simulink model "vd_controller"  (R2019b)
settings: configuration reference "E9_ECU_Configuration" (kept outside this file)
undefined symbols (not defined in the file or in its folder): BrakeMap_default_breakpoints, BrakeMap_default_data, disable_9D_front, disable_slipanglesensor, mask_select_input_pGL, Sq_PosBadGradient, Sq_PosIsFrozen, Sq_PosOutOfBounds
libraries: SignalProcessingSensorFusionLib x38, simulink x30, hdlsllib x3
(part 2 of 2)

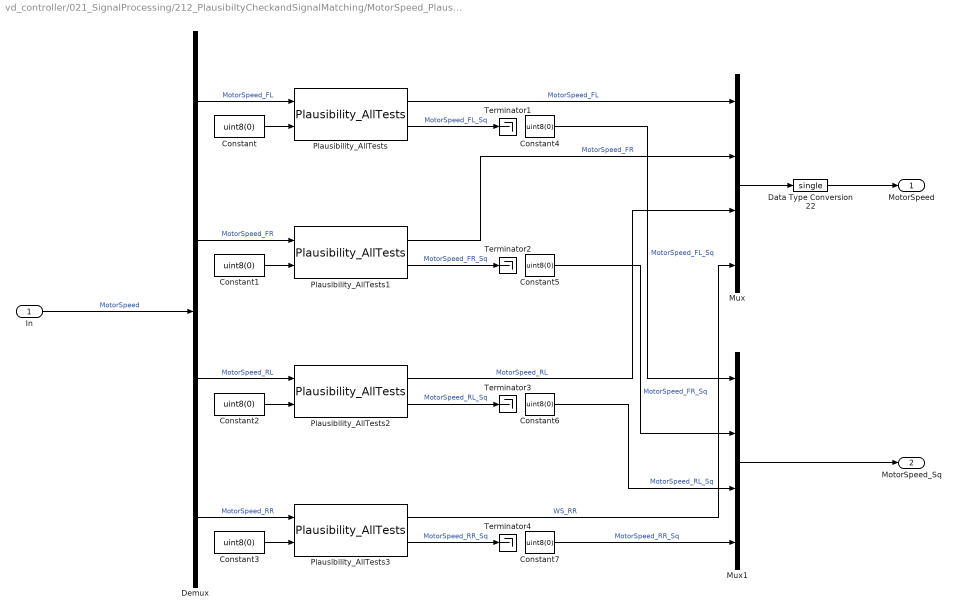
== system vd_controller/021_SignalProcessing/212_PlausibiltyCheckandSignalMatching/MotorSpeed_Plausibility ==
  In : Inport
  Constant{,1..7} (8 alike) : Constant  Value=uint8(0)
  Data Type Conversion22 : DataTypeConversion  OutDataTypeStr=single
  Demux : Demux
  Mux : Mux
  Mux1 : Mux
  Plausibility_AllTests : SignalProcessingSensorFusionLib/Plausibility_AllTests  alpha=0.4  checkGradient=off  deviation=0  threshold=0  alpha2=0  increasingPercentage=0  signalBounds=1e-10  stepDelay=40  upperBound=20000  lowerBound=-10000  useAlternativeValue=off  useManualAlternativeValue=off  manualAlternativeValue=0
  Plausibility_AllTests1 : SignalProcessingSensorFusionLib/Plausibility_AllTests  alpha=0.4  checkGradient=off  deviation=0  threshold=0  alpha2=0  increasingPercentage=0  signalBounds=1e-10  stepDelay=40  upperBound=20000  lowerBound=-10000  useAlternativeValue=off  useManualAlternativeValue=off  manualAlternativeValue=0
  Plausibility_AllTests2 : SignalProcessingSensorFusionLib/Plausibility_AllTests  alpha=0.4  checkGradient=off  deviation=0  threshold=0  alpha2=0  increasingPercentage=0  signalBounds=1e-10  stepDelay=40  upperBound=20000  lowerBound=-10000  useAlternativeValue=off  useManualAlternativeValue=off  manualAlternativeValue=0
  Plausibility_AllTests3 : SignalProcessingSensorFusionLib/Plausibility_AllTests  alpha=0  checkGradient=off  deviation=0  threshold=0  alpha2=0  increasingPercentage=0  signalBounds=1e-10  stepDelay=40  upperBound=20000  lowerBound=-10000  useAlternativeValue=off  useManualAlternativeValue=off  manualAlternativeValue=0
  Terminator{1..4} (4 alike) : Terminator
  MotorSpeed : Outport  VectorParamsAs1DForOutWhenUnconnected=off
  MotorSpeed_Sq : Outport  Port=2  VectorParamsAs1DForOutWhenUnconnected=off
  wires:
  Constant4/1 -> Mux1/1  "MotorSpeed_FL_Sq"
  Constant7/1 -> Mux1/4  "MotorSpeed_RR_Sq"
  Mux1/1 -> MotorSpeed_Sq/1
  Mux/1 -> Data Type Conversion22/1
  Plausibility_AllTests3/1 -> Mux/4  "WS_RR"
  Constant3/1 -> Plausibility_AllTests3/2
  Constant2/1 -> Plausibility_AllTests2/2
  Constant1/1 -> Plausibility_AllTests1/2
  Constant/1 -> Plausibility_AllTests/2
  Demux/4 -> Plausibility_AllTests3/1  "MotorSpeed_RR"
  Constant5/1 -> Mux1/2  "MotorSpeed_FR_Sq"
  Constant6/1 -> Mux1/3  "MotorSpeed_RL_Sq"
  Demux/3 -> Plausibility_AllTests2/1  "MotorSpeed_RL"
  Demux/2 -> Plausibility_AllTests1/1  "MotorSpeed_FR"
  Demux/1 -> Plausibility_AllTests/1  "MotorSpeed_FL"
  Plausibility_AllTests2/1 -> Mux/3  "MotorSpeed_RL"
  Plausibility_AllTests/1 -> Mux/1  "MotorSpeed_FL"
  In/1 -> Demux/1  "MotorSpeed"
  Plausibility_AllTests1/1 -> Mux/2  "MotorSpeed_FR"
  Data Type Conversion22/1 -> MotorSpeed/1
  Plausibility_AllTests/2 -> Terminator1/1  "MotorSpeed_FL_Sq"
  Plausibility_AllTests1/2 -> Terminator2/1  "MotorSpeed_FR_Sq"
  Plausibility_AllTests2/2 -> Terminator3/1  "MotorSpeed_RL_Sq"
  Plausibility_AllTests3/2 -> Terminator4/1  "MotorSpeed_RR_Sq"

== system vd_controller/021_SignalProcessing/212_PlausibiltyCheckandSignalMatching/MotorTemp_Plausibility ==
  In : Inport
  Constant{,1..3} (4 alike) : Constant  Value=uint8(0)
  Data Type Conversion{1..3,22} (4 alike) : DataTypeConversion  OutDataTypeStr=single
  Demux : Demux
  Mux : Mux
  Mux1 : Mux
  Plausibility_AllTests{,1..3} (4 alike) : SignalProcessingSensorFusionLib/Plausibility_AllTests  alpha=0.5  checkGradient=off  deviation=0  threshold=0  alpha2=0  increasingPercentage=0  signalBounds=1e-12  stepDelay=40  upperBound=250  lowerBound=-10  useAlternativeValue=off  useManualAlternativeValue=off  manualAlternativeValue=0
  MotorTempPlausible : Outport  VectorParamsAs1DForOutWhenUnconnected=off
  MotorTemp_Sq : Outport  Port=2  VectorParamsAs1DForOutWhenUnconnected=off
  wires:
  Plausibility_AllTests1/1 -> Data Type Conversion1/1  "MotorTemp_FR"
  In/1 -> Demux/1  "motorTemp"
  Plausibility_AllTests/1 -> Data Type Conversion22/1  "MotorTemp_FL"
  Plausibility_AllTests2/1 -> Data Type Conversion2/1  "MotorTemp_RL"
  Demux/1 -> Plausibility_AllTests/1
  Demux/2 -> Plausibility_AllTests1/1
  Demux/3 -> Plausibility_AllTests2/1
  Plausibility_AllTests2/2 -> Mux1/3  "MotorTemp_RL_Sq"
  Plausibility_AllTests1/2 -> Mux1/2  "MotorTemp_FR_Sq"
  Demux/4 -> Plausibility_AllTests3/1
  Constant/1 -> Plausibility_AllTests/2
  Constant1/1 -> Plausibility_AllTests1/2
  Constant2/1 -> Plausibility_AllTests2/2
  Constant3/1 -> Plausibility_AllTests3/2
  Plausibility_AllTests3/1 -> Data Type Conversion3/1  "MotorTemp_RR"
  Mux/1 -> MotorTempPlausible/1
  Mux1/1 -> MotorTemp_Sq/1
  Plausibility_AllTests3/2 -> Mux1/4  "MotorTemp_RR_Sq"
  Plausibility_AllTests/2 -> Mux1/1  "MotorTemp_Sq"
  Data Type Conversion22/1 -> Mux/1
  Data Type Conversion1/1 -> Mux/2
  Data Type Conversion2/1 -> Mux/3
  Data Type Conversion3/1 -> Mux/4

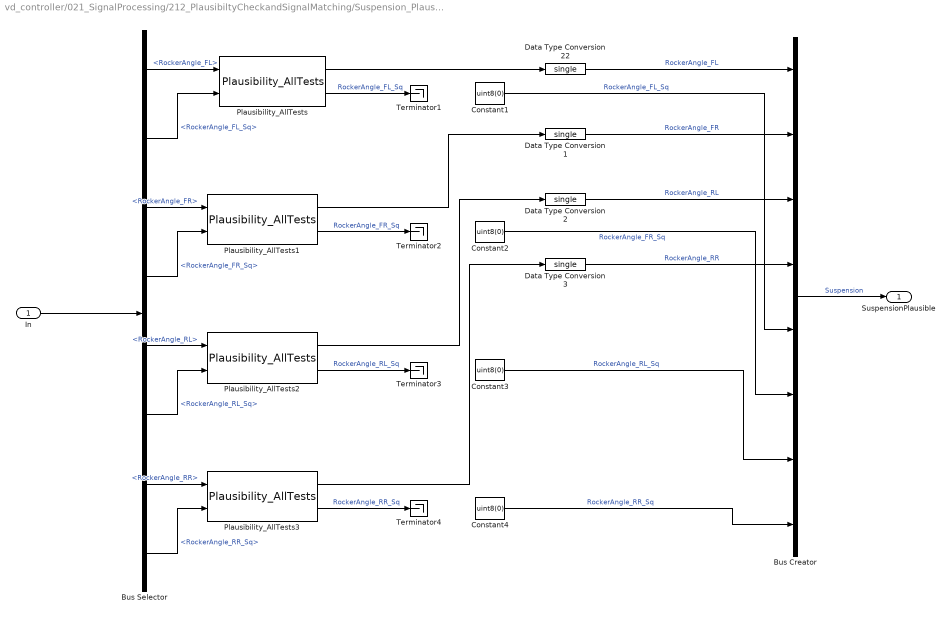
== system vd_controller/021_SignalProcessing/212_PlausibiltyCheckandSignalMatching/Suspension_Plausibility ==
  In : Inport  OutDataTypeStr=Bus: control_Suspension
  Bus Creator : BusCreator  Inputs=8  OutDataTypeStr=Bus: control_Suspension
  Bus Selector : BusSelector  OutputSignals=RockerAngle_FL,RockerAngle_FL_Sq,RockerAngle_FR,RockerAngle_FR_Sq,RockerAngle_RL,RockerAngle_RL_Sq,RockerAngle_RR,RockerAngle_RR_Sq
  Constant{1..4} (4 alike) : Constant  Value=uint8(0)
  Data Type Conversion{1..3,22} (4 alike) : DataTypeConversion  OutDataTypeStr=single
  Plausibility_AllTests{,1..3} (4 alike) : SignalProcessingSensorFusionLib/Plausibility_AllTests  alpha=0.5  checkGradient=off  deviation=0  threshold=0  alpha2=0  increasingPercentage=0  signalBounds=1e-10  stepDelay=38  upperBound=30  lowerBound=-30  useAlternativeValue=off  useManualAlternativeValue=off  manualAlternativeValue=0
  Terminator{1..4} (4 alike) : Terminator
  SuspensionPlausible : Outport  VectorParamsAs1DForOutWhenUnconnected=off
  wires:
  Constant1/1 -> Bus Creator/5  "RockerAngle_FL_Sq"
  Constant2/1 -> Bus Creator/6  "RockerAngle_FR_Sq"
  Constant3/1 -> Bus Creator/7  "RockerAngle_RL_Sq"
  Bus Selector/6 -> Plausibility_AllTests2/2  "<RockerAngle_RL_Sq>"
  Bus Selector/5 -> Plausibility_AllTests2/1  "<RockerAngle_RL>"
  Bus Selector/4 -> Plausibility_AllTests1/2  "<RockerAngle_FR_Sq>"
  Bus Selector/3 -> Plausibility_AllTests1/1  "<RockerAngle_FR>"
  Bus Selector/2 -> Plausibility_AllTests/2  "<RockerAngle_FL_Sq>"
  Bus Selector/1 -> Plausibility_AllTests/1  "<RockerAngle_FL>"
  Bus Creator/1 -> SuspensionPlausible/1  "Suspension"
  Plausibility_AllTests2/1 -> Data Type Conversion2/1
  Plausibility_AllTests/1 -> Data Type Conversion22/1
  In/1 -> Bus Selector/1
  Plausibility_AllTests1/1 -> Data Type Conversion1/1
  Bus Selector/7 -> Plausibility_AllTests3/1  "<RockerAngle_RR>"
  Constant4/1 -> Bus Creator/8  "RockerAngle_RR_Sq"
  Plausibility_AllTests3/1 -> Data Type Conversion3/1
  Bus Selector/8 -> Plausibility_AllTests3/2  "<RockerAngle_RR_Sq>"
  Data Type Conversion22/1 -> Bus Creator/1  "RockerAngle_FL"
  Data Type Conversion1/1 -> Bus Creator/2  "RockerAngle_FR"
  Data Type Conversion2/1 -> Bus Creator/3  "RockerAngle_RL"
  Data Type Conversion3/1 -> Bus Creator/4  "RockerAngle_RR"
  Plausibility_AllTests/2 -> Terminator1/1  "RockerAngle_FL_Sq"
  Plausibility_AllTests1/2 -> Terminator2/1  "RockerAngle_FR_Sq"
  Plausibility_AllTests2/2 -> Terminator3/1  "RockerAngle_RL_Sq"
  Plausibility_AllTests3/2 -> Terminator4/1  "RockerAngle_RR_Sq"

== system vd_controller/021_SignalProcessing/212_PlausibiltyCheckandSignalMatching/WheelSpeed_Plausibility ==
  note: Dieser Block ist eigentlich überflüssig. Der Zusammenhang von MotorSpeed und WheelSpeed ist sehr simpel (selbe Messgröße).
      | Es reicht aus, nur diePlausibilität von MotorSpeed zu prüfen und daraufhin MotorSpeed und WheelSpeed gleichzeitig zu bewerten.
  In : Inport
  Constant{,1..3} (4 alike) : Constant  Value=uint8(0)
  Data Type Conversion{1..3,22} (4 alike) : DataTypeConversion  OutDataTypeStr=single
  Demux : Demux
  Mux : Mux
  Mux1 : Mux
  Plausibility_AllTests{,1..3} (4 alike) : SignalProcessingSensorFusionLib/Plausibility_AllTests  alpha=0.3  checkGradient=off  deviation=0  threshold=0  alpha2=0  increasingPercentage=0  signalBounds=1e-12  stepDelay=40  upperBound=100  lowerBound=-10  useAlternativeValue=off  useManualAlternativeValue=off  manualAlternativeValue=0
  WheelSpeedPlausible : Outport  VectorParamsAs1DForOutWhenUnconnected=off
  WheelSpeed_Sq : Outport  Port=2  VectorParamsAs1DForOutWhenUnconnected=off
  wires:
  Plausibility_AllTests1/1 -> Data Type Conversion1/1  "WheelSpeed_FR"
  In/1 -> Demux/1  "wheelSpeed"
  Plausibility_AllTests/1 -> Data Type Conversion22/1  "WheelSpeed_FL"
  Plausibility_AllTests2/1 -> Data Type Conversion2/1  "WheelSpeed_RL"
  Demux/1 -> Plausibility_AllTests/1  "WheelSpeed_FL"
  Demux/2 -> Plausibility_AllTests1/1  "WheelSpeed_FR"
  Demux/3 -> Plausibility_AllTests2/1  "WheelSpeed_RL"
  Plausibility_AllTests2/2 -> Mux1/3  "WheelSpeed_RL_Sq"
  Plausibility_AllTests1/2 -> Mux1/2  "WheelSpeed_FR_Sq"
  Demux/4 -> Plausibility_AllTests3/1  "WheelSpeed_RR"
  Constant/1 -> Plausibility_AllTests/2
  Constant1/1 -> Plausibility_AllTests1/2
  Constant2/1 -> Plausibility_AllTests2/2
  Constant3/1 -> Plausibility_AllTests3/2
  Plausibility_AllTests3/1 -> Data Type Conversion3/1  "WheelSpeed_RR"
  Mux/1 -> WheelSpeedPlausible/1
  Mux1/1 -> WheelSpeed_Sq/1
  Plausibility_AllTests3/2 -> Mux1/4  "WheelSpeed_RR_Sq"
  Plausibility_AllTests/2 -> Mux1/1  "WheelSpeed_FL_Sq"
  Data Type Conversion22/1 -> Mux/1
  Data Type Conversion1/1 -> Mux/2
  Data Type Conversion2/1 -> Mux/3
  Data Type Conversion3/1 -> Mux/4

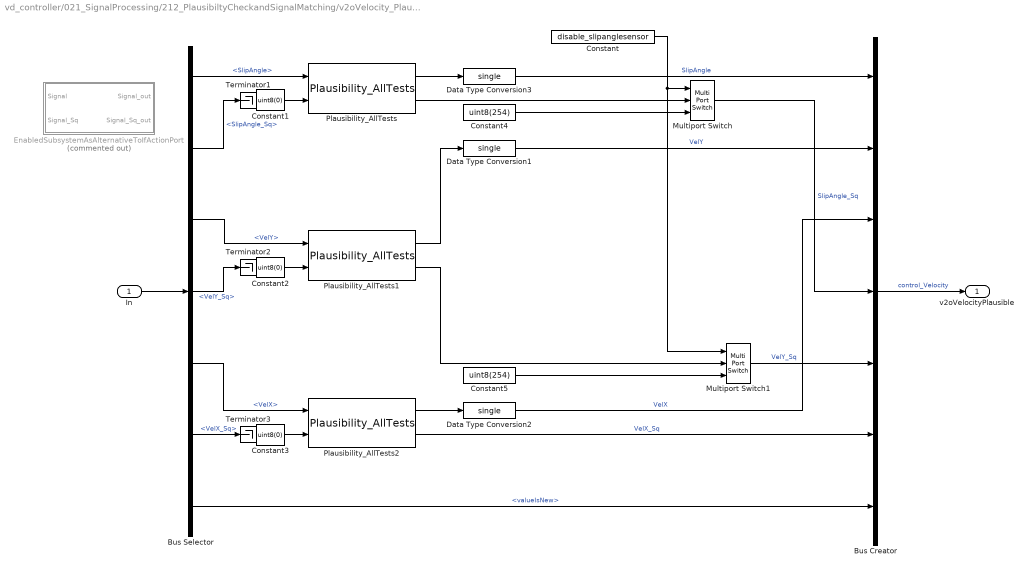
== system vd_controller/021_SignalProcessing/212_PlausibiltyCheckandSignalMatching/v2oVelocity_Plausibility ==
  In : Inport  OutDataTypeStr=Bus: control_Velocity
  Bus Creator : BusCreator  Inputs=7  OutDataTypeStr=Bus: control_Velocity
  Bus Selector : BusSelector  OutputSignals=SlipAngle,SlipAngle_Sq,VelY,VelY_Sq,VelX,VelX_Sq,valueIsNew
  Constant : Constant  Value=disable_slipanglesensor
  Constant1 : Constant  Value=uint8(0)
  Constant2 : Constant  Value=uint8(0)
  Constant3 : Constant  Value=uint8(0)
  Constant4 : Constant  Value=uint8(254)
  Constant5 : Constant  Value=uint8(254)
  Data Type Conversion1 : DataTypeConversion  OutDataTypeStr=single
  Data Type Conversion2 : DataTypeConversion  OutDataTypeStr=single
  Data Type Conversion3 : DataTypeConversion  OutDataTypeStr=single
  EnabledSubsystemAsAlternativeToIfActionPort : Subsystem  Commented=on  AncestorBlock=SignalProcessingSensorFusionLib/Plausibility_AllTests  mask{alpha=0.3, checkGradient=off, deviation=0, threshold=0, alpha2=0, increasingPercentage=0, signalBounds=1e-8, stepDelay=35, upperBound=90, lowerBound=-90, useAlternativeValue=off, useManualAlternativeValue=off, manualAlternativeValue=0}
      mask prompts: alpha "alpha-value"; checkGradient "Shall the gradient be controlled?"; deviation "gain for accepted deviation"; threshold "Maximal Change per Second"; alpha2 "Inertia of mean (0-1)"; increasingPercentage "percent of the max. changerate add to the allowed deviation [%]"; signalBounds "Signal Bounds"; stepDelay "Step Delay"; upperBound "upper bound"; lowerBound "lower bound"; useAlternativeValue "Shall a alternative value be used if signal is not plausible?"; useManualAlternativeValue "Shall a manually given Value be used? Otherwise signal is held."; manualAlternativeValue "manually given Value"
      mask DialogControl LowPassSettings Prompt: lowpass
      mask DialogControl BadGradientSettings Prompt: bad gradient
      mask DialogControl increasingPercentage Tooltip: How many percent of the max. Change per Second the allowed deviation rises
      mask DialogControl Container8 Prompt: frozen value
      mask DialogControl signalBounds Tooltip: (in which bounds consecutive singals can differ to be detected as frozen )
      mask DialogControl stepDelay Tooltip: how many steps the singal must be within the bounds, so that the signal is detected as frozen
      mask DialogControl Bounds Prompt: bounds
      mask DialogControl AlternativeValue Prompt: alternative Value
      mask DialogControl Container12 Prompt: Use manually given Value
  Multiport Switch : MultiPortSwitch  DataPortOrder=Zero-based contiguous  Inputs=2  zeroidx=on
  Multiport Switch1 : MultiPortSwitch  DataPortOrder=Zero-based contiguous  Inputs=2  zeroidx=on
  Plausibility_AllTests : SignalProcessingSensorFusionLib/Plausibility_AllTests  alpha=0.3  checkGradient=off  deviation=0  threshold=0  alpha2=0  increasingPercentage=0  signalBounds=1e-8  stepDelay=35  upperBound=90  lowerBound=-90  useAlternativeValue=off  useManualAlternativeValue=off  manualAlternativeValue=0
  Plausibility_AllTests1 : SignalProcessingSensorFusionLib/Plausibility_AllTests  alpha=0.3  checkGradient=off  deviation=0  threshold=0  alpha2=0  increasingPercentage=0  signalBounds=1e-8  stepDelay=35  upperBound=50  lowerBound=-50  useAlternativeValue=off  useManualAlternativeValue=off  manualAlternativeValue=0
  Plausibility_AllTests2 : SignalProcessingSensorFusionLib/Plausibility_AllTests  alpha=0.5  checkGradient=off  deviation=0  threshold=0  alpha2=0  increasingPercentage=0  signalBounds=1e-8  stepDelay=35  upperBound=36  lowerBound=-3  useAlternativeValue=off  useManualAlternativeValue=off  manualAlternativeValue=0
  Terminator1 : Terminator
  Terminator2 : Terminator
  Terminator3 : Terminator
  v2oVelocityPlausible : Outport  VectorParamsAs1DForOutWhenUnconnected=off
  wires:
  Plausibility_AllTests1/1 -> Data Type Conversion1/1
  In/1 -> Bus Selector/1
  Plausibility_AllTests/1 -> Data Type Conversion3/1
  Plausibility_AllTests2/1 -> Data Type Conversion2/1
  Bus Creator/1 -> v2oVelocityPlausible/1  "control_Velocity"
  Bus Selector/1 -> Plausibility_AllTests/1  "<SlipAngle>"
  Bus Selector/2 -> Terminator1/1  "<SlipAngle_Sq>"
  Bus Selector/3 -> Plausibility_AllTests1/1  "<VelY>"
  Bus Selector/4 -> Terminator2/1  "<VelY_Sq>"
  Bus Selector/5 -> Plausibility_AllTests2/1  "<VelX>"
  Bus Selector/6 -> Terminator3/1  "<VelX_Sq>"
  Bus Selector/7 -> Bus Creator/7  "<valueIsNew>"
  Data Type Conversion1/1 -> Bus Creator/2  "VelY"
  Data Type Conversion3/1 -> Bus Creator/1  "SlipAngle"
  Data Type Conversion2/1 -> Bus Creator/3  "VelX"
  Plausibility_AllTests/2 -> Multiport Switch/2
  Plausibility_AllTests1/2 -> Multiport Switch1/2
  Plausibility_AllTests2/2 -> Bus Creator/6  "VelX_Sq"
  Constant1/1 -> Plausibility_AllTests/2
  Constant2/1 -> Plausibility_AllTests1/2
  Constant3/1 -> Plausibility_AllTests2/2
  Constant/1 -> Multiport Switch1/1, Multiport Switch/1
  Constant4/1 -> Multiport Switch/3
  Multiport Switch1/1 -> Bus Creator/5  "VelY_Sq"
  Constant5/1 -> Multiport Switch1/3
  Multiport Switch/1 -> Bus Creator/4  "SlipAngle_Sq"

== system vd_controller/021_SignalProcessing/214_ManualMode and SimInput/9DFront ==
  Signal_In : Inport
  Enable : Inport  Port=2
  Bitwise Operator : simulink/Logic and Bit Operations/Bitwise Operator  logicop=AND  UseBitMask=on  BitMask=bin2dec('11011001')  BitMaskRealWorld=Stored Integer
  Sinus-schwingung : Subsystem  Commented=on
  Switch : Switch  Criteria=u2 ~= 0  Threshold=U2==0
  9DFront : Outport  VectorParamsAs1DForOutWhenUnconnected=off
  wires:
  Bitwise Operator/1 -> Switch/2
  Signal_In/1 -> Switch/1, Switch/3  "9DFront"
  Enable/1 -> Bitwise Operator/1
  Switch/1 -> 9DFront/1  "9DFront"

== system vd_controller/021_SignalProcessing/214_ManualMode and SimInput/9DRear ==
  Signal_In : Inport
  Enable : Inport  Port=2
  Bitwise Operator : simulink/Logic and Bit Operations/Bitwise Operator  logicop=AND  UseBitMask=on  BitMask=bin2dec('11011001')  BitMaskRealWorld=Stored Integer
  Constant : Constant
  Constant1 : Constant
  Switch : Switch  Criteria=u2 ~= 0  Threshold=U2==0
  Terminator : Terminator
  9DRear : Outport  VectorParamsAs1DForOutWhenUnconnected=off
  wires:
  Enable/1 -> Bitwise Operator/1
  Signal_In/1 -> 9DRear/1  "9DRear"
  Bitwise Operator/1 -> Switch/2
  Constant/1 -> Switch/1
  Constant1/1 -> Switch/3
  Switch/1 -> Terminator/1  "9DRear"

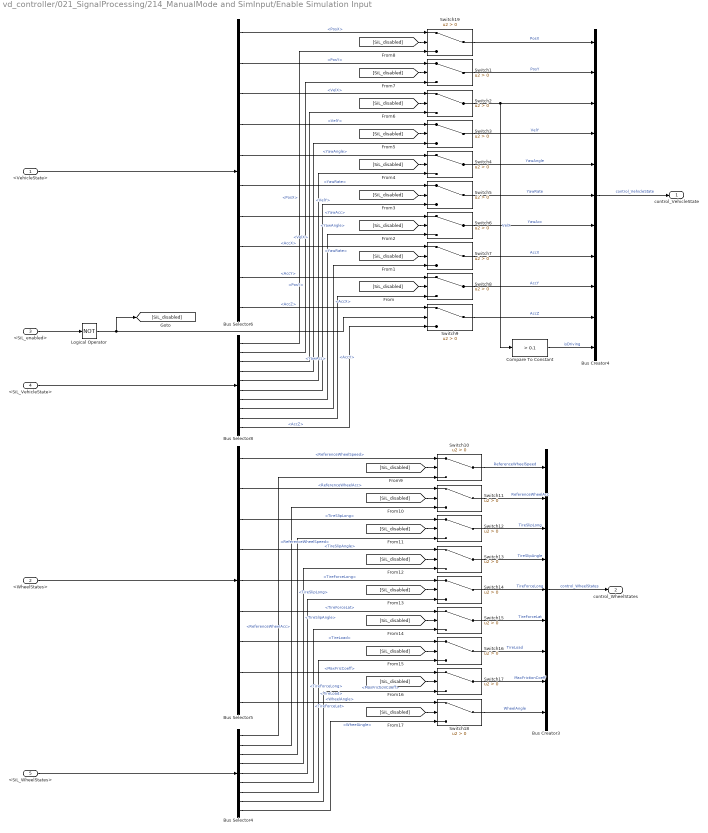
== system vd_controller/021_SignalProcessing/214_ManualMode and SimInput/Enable Simulation Input ==
  <VehicleState> : Inport
  <WheelStates> : Inport  Port=2
  <SiL_enabled> : Inport  Port=3
  <SiL_VehicleState> : Inport  Port=4
  <SiL_WheelStates> : Inport  Port=5
  Bus Creator3 : BusCreator  Inputs=9  OutDataTypeStr=Bus: control_WheelStates
  Bus Creator4 : BusCreator  Inputs=11  OutDataTypeStr=Bus: control_VehicleState
  Bus Selector4 : BusSelector  OutputSignals=ReferenceWheelSpeed,ReferenceWheelAcc,TireSlipLong,TireSlipAngle,TireForceLong,TireForceLat,TireLoad,MaxFrictionCoeff,WheelAngle
  Bus Selector5 : BusSelector  OutputSignals=ReferenceWheelSpeed,ReferenceWheelAcc,TireSlipLong,TireSlipAngle,TireForceLong,TireForceLat,TireLoad,MaxFricCoeff,WheelAngle
  Bus Selector6 : BusSelector  OutputSignals=PosX,PosY,VelX,VelY,YawAngle,YawRate,YawAcc,AccX,AccY,AccZ
  Bus Selector8 : BusSelector  OutputSignals=PosX,PosY,VelX,VelY,YawAngle,YawRate,YawAcc,AccX,AccY,AccZ
  Compare To Constant : simulink/Logic and Bit Operations/Compare To Constant  relop=>  const=0.1  OutDataTypeStr=boolean
  Logical Operator : Logic  Operator=NOT  AllPortsSameDT=off  OutDataTypeStr=boolean
  Switch{1..19} (19 alike) : Switch  Criteria=u2 > Threshold
  control_VehicleState : Outport  VectorParamsAs1DForOutWhenUnconnected=off
  control_WheelStates : Outport  Port=2  VectorParamsAs1DForOutWhenUnconnected=off
  wires:
  Bus Selector8/3 -> Switch2/3  "<VelX>"
  Switch3/1 -> Bus Creator4/4  "VelY"
  <SiL_enabled>/1 -> Logical Operator/1
  Bus Selector8/8 -> Switch7/3  "<AccX>"
  Switch17/1 -> Bus Creator3/8  "MaxFrictionCoeff"
  Bus Selector5/1 -> Switch10/1  "<ReferenceWheelSpeed>"
  Bus Selector5/8 -> Switch17/1  "<MaxFricCoeff>"
  Bus Selector5/4 -> Switch13/1  "<TireSlipAngle>"
  Switch12/1 -> Bus Creator3/3  "TireSlipLong"
  Bus Selector8/9 -> Switch8/3  "<AccY>"
  Bus Selector8/6 -> Switch5/3  "<YawRate>"
  Bus Creator4/1 -> control_VehicleState/1  "control_VehicleState"
  Bus Selector5/2 -> Switch11/1  "<ReferenceWheelAcc>"
  Switch4/1 -> Bus Creator4/5  "YawAngle"
  Bus Selector8/4 -> Switch3/3  "<VelY>"
  Switch14/1 -> Bus Creator3/5  "TireForceLong"
  Switch6/1 -> Bus Creator4/7  "YawAcc"
  Bus Selector5/9 -> Switch18/1  "<WheelAngle>"
  Bus Selector8/5 -> Switch4/3  "<YawAngle>"
  Switch2/1 -> Compare To Constant/1, Bus Creator4/3  "VelX"
  Switch18/1 -> Bus Creator3/9  "WheelAngle"
  Bus Selector5/7 -> Switch16/1  "<TireLoad>"
  Bus Selector5/5 -> Switch14/1  "<TireForceLong>"
  <WheelStates>/1 -> Bus Selector5/1
  Switch10/1 -> Bus Creator3/1  "ReferenceWheelSpeed"
  Bus Selector8/7 -> Switch6/3  "<YawAcc>"
  Switch7/1 -> Bus Creator4/8  "AccX"
  Switch11/1 -> Bus Creator3/2  "ReferenceWheelAcc"
  Switch13/1 -> Bus Creator3/4  "TireSlipAngle"
  Switch8/1 -> Bus Creator4/9  "AccY"
  Bus Selector6/1 -> Switch19/1  "<PosX>"
  Switch19/1 -> Bus Creator4/1  "PosX"
  Bus Selector5/6 -> Switch15/1  "<TireForceLat>"
  Bus Creator3/1 -> control_WheelStates/1  "control_WheelStates"
  Switch16/1 -> Bus Creator3/7  "TireLoad"
  Switch5/1 -> Bus Creator4/6  "YawRate"
  Switch1/1 -> Bus Creator4/2  "PosY"
  Switch15/1 -> Bus Creator3/6  "TireForceLat"
  Bus Selector5/3 -> Switch12/1  "<TireSlipLong>"
  Switch9/1 -> Bus Creator4/10  "AccZ"
  Bus Selector8/10 -> Switch9/3  "<AccZ>"
  <SiL_VehicleState>/1 -> Bus Selector8/1
  <SiL_WheelStates>/1 -> Bus Selector4/1
  <VehicleState>/1 -> Bus Selector6/1
  Bus Selector6/2 -> Switch1/1  "<PosY>"
  Logical Operator/1 -> Switch9/2, [SiL_disabled]
  Bus Selector6/3 -> Switch2/1  "<VelX>"
  Bus Selector6/4 -> Switch3/1  "<VelY>"
  Bus Selector6/5 -> Switch4/1  "<YawAngle>"
  Bus Selector6/6 -> Switch5/1  "<YawRate>"
  Bus Selector6/7 -> Switch6/1  "<YawAcc>"
  Bus Selector6/8 -> Switch7/1  "<AccX>"
  Bus Selector6/9 -> Switch8/1  "<AccY>"
  Bus Selector6/10 -> Switch9/1  "<AccZ>"
  [SiL_disabled] -> Switch8/2
  [SiL_disabled] -> Switch7/2
  [SiL_disabled] -> Switch6/2
  [SiL_disabled] -> Switch5/2
  [SiL_disabled] -> Switch4/2
  [SiL_disabled] -> Switch3/2
  [SiL_disabled] -> Switch2/2
  [SiL_disabled] -> Switch1/2
  [SiL_disabled] -> Switch19/2
  Bus Selector8/1 -> Switch19/3  "<PosX>"
  Bus Selector8/2 -> Switch1/3  "<PosY>"
  [SiL_disabled] -> Switch10/2
  [SiL_disabled] -> Switch11/2
  [SiL_disabled] -> Switch12/2
  [SiL_disabled] -> Switch13/2
  [SiL_disabled] -> Switch14/2
  [SiL_disabled] -> Switch15/2
  [SiL_disabled] -> Switch16/2
  [SiL_disabled] -> Switch17/2
  [SiL_disabled] -> Switch18/2
  Bus Selector4/1 -> Switch10/3  "<ReferenceWheelSpeed>"
  Bus Selector4/2 -> Switch11/3  "<ReferenceWheelAcc>"
  Bus Selector4/3 -> Switch12/3  "<TireSlipLong>"
  Bus Selector4/4 -> Switch13/3  "<TireSlipAngle>"
  Bus Selector4/5 -> Switch14/3  "<TireForceLong>"
  Bus Selector4/6 -> Switch15/3  "<TireForceLat>"
  Bus Selector4/7 -> Switch16/3  "<TireLoad>"
  Bus Selector4/8 -> Switch17/3  "<MaxFrictionCoeff>"
  Bus Selector4/9 -> Switch18/3  "<WheelAngle>"
  Compare To Constant/1 -> Bus Creator4/11  "isDriving"

== system vd_controller/021_SignalProcessing/214_ManualMode and SimInput/HMI_DriverNotice ==
  Signal_In : Inport
  Enable : Inport  Port=2
  Bitwise Operator : simulink/Logic and Bit Operations/Bitwise Operator  Commented=on  logicop=AND  UseBitMask=on  BitMask=bin2dec('11011001')  BitMaskRealWorld=Stored Integer
  Constant : Constant  Commented=on
  Switch : Switch  Commented=on  Criteria=u2 ~= 0  Threshold=U2==0
  Terminator : Terminator
  HMI_DriverNotice : Outport  VectorParamsAs1DForOutWhenUnconnected=off
  wires:
  Bitwise Operator/1 -> Switch/2
  Signal_In/1 -> HMI_DriverNotice/1  "HMI_DriverNotice"
  Enable/1 -> Bitwise Operator/1
  Constant/1 -> Switch/1
  Switch/1 -> Terminator/1  "HMI_DriverNotice"

== system vd_controller/021_SignalProcessing/214_ManualMode and SimInput/electric ==
  Signal_In : Inport
  Enable : Inport  Port=2
  Bitwise Operator : simulink/Logic and Bit Operations/Bitwise Operator  logicop=AND  UseBitMask=on  BitMask=bin2dec('11011001')  BitMaskRealWorld=Stored Integer
  Constant : Constant
  Constant1 : Constant
  Switch : Switch  Criteria=u2 ~= 0  Threshold=U2==0
  Terminator : Terminator
  electric : Outport  VectorParamsAs1DForOutWhenUnconnected=off
  wires:
  Signal_In/1 -> electric/1  "electric"
  Bitwise Operator/1 -> Switch/2
  Enable/1 -> Bitwise Operator/1
  Constant1/1 -> Switch/3
  Switch/1 -> Terminator/1  "9DRear"
  Constant/1 -> Switch/1

== system vd_controller/021_SignalProcessing/214_ManualMode and SimInput/inverterTemp ==
  Signal_In : Inport
  Enable : Inport  Port=2
  Bitwise Operator : simulink/Logic and Bit Operations/Bitwise Operator  logicop=AND  UseBitMask=on  BitMask=bin2dec('11011001')  BitMaskRealWorld=Stored Integer
  Constant : Constant  OutDataTypeStr=single
  Switch : Switch  Criteria=u2 ~= 0  Threshold=U2==0  OutDataTypeStr=single
  inverterTemp : Outport  OutDataTypeStr=single  PortDimensions=4  VectorParamsAs1DForOutWhenUnconnected=off
  wires:
  Signal_In/1 -> Switch/3
  Enable/1 -> Bitwise Operator/1
  Switch/1 -> inverterTemp/1  "inverterTemp"
  Bitwise Operator/1 -> Switch/2
  Constant/1 -> Switch/1

== system vd_controller/021_SignalProcessing/214_ManualMode and SimInput/motorSpeed ==
  Signal_In : Inport
  Enable : Inport  Port=2
  Bitwise Operator : simulink/Logic and Bit Operations/Bitwise Operator  logicop=AND  UseBitMask=on  BitMask=bin2dec('11011001')  BitMaskRealWorld=Stored Integer
  Constant : Constant  Value=[1;1;1;1]  OutDataTypeStr=Inherit: Inherit via back propagation
  Switch : Switch  Criteria=u2 ~= 0  Threshold=U2==0
  motorSpeed : Outport  VectorParamsAs1DForOutWhenUnconnected=off
  wires:
  Bitwise Operator/1 -> Switch/2
  Switch/1 -> motorSpeed/1  "motorSpeed"
  Enable/1 -> Bitwise Operator/1
  Signal_In/1 -> Switch/3
  Constant/1 -> Switch/1

== system vd_controller/021_SignalProcessing/214_ManualMode and SimInput/motorTemp ==
  Signal_In : Inport
  Enable : Inport  Port=2
  Bitwise Operator : simulink/Logic and Bit Operations/Bitwise Operator  logicop=AND  UseBitMask=on  BitMask=bin2dec('11011001')  BitMaskRealWorld=Stored Integer
  Constant : Constant  OutDataTypeStr=single
  Switch : Switch  Criteria=u2 ~= 0  Threshold=U2==0  OutDataTypeStr=single
  motorTemp : Outport  OutDataTypeStr=single  PortDimensions=4  VectorParamsAs1DForOutWhenUnconnected=off
  wires:
  Bitwise Operator/1 -> Switch/2
  Switch/1 -> motorTemp/1  "motorTemp"
  Enable/1 -> Bitwise Operator/1
  Signal_In/1 -> Switch/3
  Constant/1 -> Switch/1

== system vd_controller/021_SignalProcessing/214_ManualMode and SimInput/settings ==
  Signal_In : Inport
  Enable : Inport  Port=2
  Bitwise Operator : simulink/Logic and Bit Operations/Bitwise Operator  logicop=AND  UseBitMask=on  BitMask=bin2dec('11011001')  BitMaskRealWorld=Stored Integer
  Constant : Constant
  Constant1 : Constant
  Switch : Switch  Criteria=u2 ~= 0  Threshold=U2==0
  Terminator : Terminator
  settings : Outport  VectorParamsAs1DForOutWhenUnconnected=off
  wires:
  Bitwise Operator/1 -> Switch/2
  Signal_In/1 -> settings/1  "settings"
  Enable/1 -> Bitwise Operator/1
  Constant1/1 -> Switch/3
  Constant/1 -> Switch/1
  Switch/1 -> Terminator/1  "settings"

== system vd_controller/021_SignalProcessing/214_ManualMode and SimInput/suspHall ==
  Signal_In : Inport
  Enable : Inport  Port=2
  Bitwise Operator : simulink/Logic and Bit Operations/Bitwise Operator  logicop=AND  UseBitMask=on  BitMask=bin2dec('11011001')  BitMaskRealWorld=Stored Integer
  Constant : Constant
  Constant1 : Constant
  Switch : Switch  Criteria=u2 ~= 0  Threshold=U2==0
  Terminator : Terminator
  suspHall : Outport  VectorParamsAs1DForOutWhenUnconnected=off
  wires:
  Signal_In/1 -> suspHall/1
  Constant1/1 -> Switch/3
  Enable/1 -> Bitwise Operator/1
  Switch/1 -> Terminator/1  "9DRear"
  Bitwise Operator/1 -> Switch/2
  Constant/1 -> Switch/1

== system vd_controller/021_SignalProcessing/214_ManualMode and SimInput/v2oVelocity ==
  Signal_In : Inport
  Enable : Inport  Port=2
  Bitwise Operator : simulink/Logic and Bit Operations/Bitwise Operator  logicop=AND  UseBitMask=on  BitMask=bin2dec('11011001')  BitMaskRealWorld=Stored Integer
  Constant : Constant
  Constant1 : Constant
  Switch : Switch  Criteria=u2 ~= 0  Threshold=U2==0
  Terminator : Terminator
  v2oVelocity : Outport  VectorParamsAs1DForOutWhenUnconnected=off
  wires:
  Signal_In/1 -> v2oVelocity/1  "v2oVelocity"
  Constant1/1 -> Switch/3
  Enable/1 -> Bitwise Operator/1
  Switch/1 -> Terminator/1  "9DRear"
  Bitwise Operator/1 -> Switch/2
  Constant/1 -> Switch/1

== system vd_controller/021_SignalProcessing/214_ManualMode and SimInput/wheelSpeed ==
  Signal_In : Inport
  Enable : Inport  Port=2
  Bitwise Operator : simulink/Logic and Bit Operations/Bitwise Operator  logicop=AND  UseBitMask=on  BitMask=bin2dec('11011001')  BitMaskRealWorld=Stored Integer
  Constant : Constant
  Constant1 : Constant
  Switch : Switch  Criteria=u2 ~= 0  Threshold=U2==0
  Terminator : Terminator
  wheelSpeed : Outport  VectorParamsAs1DForOutWhenUnconnected=off
  wires:
  Signal_In/1 -> wheelSpeed/1  "wheelSpeed"
  Constant1/1 -> Switch/3
  Enable/1 -> Bitwise Operator/1
  Switch/1 -> Terminator/1  "9DRear"
  Bitwise Operator/1 -> Switch/2
  Constant/1 -> Switch/1

== system vd_controller/021_SignalProcessing/214_ManualMode and SimInput/wheelTorque ==
  Signal_In : Inport
  Enable : Inport  Port=2
  Bitwise Operator : simulink/Logic and Bit Operations/Bitwise Operator  logicop=AND  UseBitMask=on  BitMask=bin2dec('11011001')  BitMaskRealWorld=Stored Integer
  Constant : Constant
  Constant1 : Constant
  Switch : Switch  Criteria=u2 ~= 0  Threshold=U2==0
  Terminator : Terminator
  wheelTorque : Outport  VectorParamsAs1DForOutWhenUnconnected=off
  wires:
  Signal_In/1 -> wheelTorque/1
  Constant/1 -> Switch/1
  Constant1/1 -> Switch/3
  Bitwise Operator/1 -> Switch/2
  Enable/1 -> Bitwise Operator/1
  Switch/1 -> Terminator/1  "9DRear"

== system vd_controller/021_SignalProcessing/211_DriverSignalProcessing/DriverDemand_Generation_LaunchControl/Brake Map ==
  note: Bitte mit den Kennlinien unterhalb der 45 Grad Ursprungsgeraden bleiben, Einfluss auf die PowerLimitation sonst nicht auszuschließen
  note: Verschiedene Standard-Pedalmappings (ohne Geschwindigkeits- und Bremskraftfaktoreinfluss) für unterschiedliche Fahrer
  BrakeTorque : Inport
  Driver : Inport  Port=2
  AlDe : Lookup_n-D  NumberOfTableDimensions=1  BreakpointsForDimension1=[0:0.1:1]  Table=[0:0.1:1]  InternalRulePriority=Speed  RndMeth=Simplest  InputSameDT=on
  FeSch : Lookup_n-D  NumberOfTableDimensions=1  BreakpointsForDimension1=[0:0.1:1]  Table=[0:0.1:1]  InternalRulePriority=Speed  RndMeth=Simplest  InputSameDT=on
  Multiport Switch : MultiPortSwitch  DataPortOrder=Zero-based contiguous  Inputs=4  zeroidx=on
  SiRi : Lookup_n-D  NumberOfTableDimensions=1  BreakpointsForDimension1=[0:0.1:1]  Table=[0:0.1:1]  InternalRulePriority=Speed  RndMeth=Simplest  InputSameDT=on
  default : Lookup_n-D  NumberOfTableDimensions=1  BreakpointsForDimension1=BrakeMap_default_breakpoints  Table=BrakeMap_default_data  InternalRulePriority=Speed  RndMeth=Simplest  InputSameDT=on
  DriverBrakeTorque : Outport  VectorParamsAs1DForOutWhenUnconnected=off
  wires:
  default/1 -> Multiport Switch/2
  Multiport Switch/1 -> DriverBrakeTorque/1  "DriverBrakeTorque"
  BrakeTorque/1 -> default/1, AlDe/1, SiRi/1, FeSch/1
  FeSch/1 -> Multiport Switch/4
  AlDe/1 -> Multiport Switch/3
  SiRi/1 -> Multiport Switch/5
  Driver/1 -> Multiport Switch/1

== system vd_controller/021_SignalProcessing/211_DriverSignalProcessing/DriverDemand_Generation_LaunchControl/Subsystem ==
  Drive Request : Inport
  DrivingMode : Inport  Port=2
  DriverDemand_z : Inport  Port=3
  "Aktiviere AccelPedalLogic nur in AccelModus " : simulink/Logic and Bit Operations/Compare To Constant  relop===  const=3  OutDataTypeStr=boolean
  EntryBedingung für AccelPedalLogic : simulink/Logic and Bit Operations/Compare To Constant  relop===  const=1  OutDataTypeStr=boolean
  LeaveBedingung für AccelPedalLogic : simulink/Logic and Bit Operations/Compare To Constant  relop=>=  const=0.5  OutDataTypeStr=boolean
  Logical Operator : Logic  Inputs=3  AllPortsSameDT=off  OutDataTypeStr=boolean
  AccelPedalEnable : Outport  VectorParamsAs1DForOutWhenUnconnected=off
  wires:
  EntryBedingung für AccelPedalLogic/1 -> Logical Operator/3
  LeaveBedingung für AccelPedalLogic/1 -> Logical Operator/1
  Logical Operator/1 -> AccelPedalEnable/1  "AccelPedalEnable"
  DrivingMode/1 -> "Aktiviere AccelPedalLogic nur in AccelModus "/1
  "Aktiviere AccelPedalLogic nur in AccelModus "/1 -> Logical Operator/2
  DriverDemand_z/1 -> EntryBedingung für AccelPedalLogic/1
  Drive Request/1 -> LeaveBedingung für AccelPedalLogic/1

== system vd_controller/021_SignalProcessing/211_DriverSignalProcessing/DriverDemand_Generation_LaunchControl/Totbereich Bremspedal ==
  note: Totbereich Pedale
  Pedal_BrakeRecu_Value : Inport
  Gain1 : Gain
  Kompensation auf ursprünglichen Wertebereich : Gain  Gain=1/0.95
  Totzone Bremspedal : DeadZone  LowerValue=0  UpperValue=0.05  SaturateOnIntegerOverflow=on
  maximaler Wert durch Totzone : Saturate  UpperLimit=0.95  LowerLimit=0
  BrakeTorque : Outport  VectorParamsAs1DForOutWhenUnconnected=off
  wires:
  Pedal_BrakeRecu_Value/1 -> Gain1/1
  maximaler Wert durch Totzone/1 -> Kompensation auf ursprünglichen Wertebereich/1
  Kompensation auf ursprünglichen Wertebereich/1 -> BrakeTorque/1  "BrakeTorque"
  Totzone Bremspedal/1 -> maximaler Wert durch Totzone/1
  Gain1/1 -> Totzone Bremspedal/1  "BrakeReq"

== system vd_controller/021_SignalProcessing/211_DriverSignalProcessing/DriverDemand_Generation_LaunchControl/Totbereich Gaspedal ==
  Pedal_Accel_Value : Inport
  Gain : Gain
  Kompensation auf ursprünglichen Wertebereich : Gain  Gain=1/0.98
  To Drive Torque : Gain
  Totzone Gaspedal : DeadZone  LowerValue=0  UpperValue=0.02  SaturateOnIntegerOverflow=on
  maximaler Wert durch Totzone : Saturate  UpperLimit=0.98  LowerLimit=0
  Drive Request : Outport  VectorParamsAs1DForOutWhenUnconnected=off
  wires:
  Totzone Gaspedal/1 -> maximaler Wert durch Totzone/1
  Gain/1 -> Totzone Gaspedal/1  "TorqueReq"
  maximaler Wert durch Totzone/1 -> Kompensation auf ursprünglichen Wertebereich/1
  To Drive Torque/1 -> Drive Request/1  "Drive Request"
  Pedal_Accel_Value/1 -> Gain/1
  Kompensation auf ursprünglichen Wertebereich/1 -> To Drive Torque/1

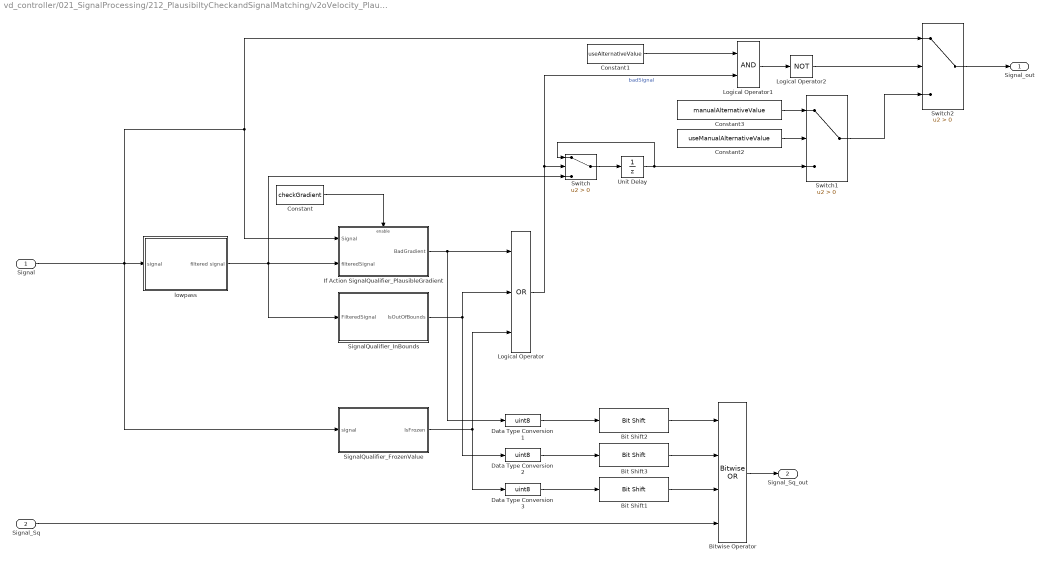
== system vd_controller/021_SignalProcessing/212_PlausibiltyCheckandSignalMatching/v2oVelocity_Plausibility/EnabledSubsystemAsAlternativeToIfActionPort ==
  Signal : Inport
  Signal_Sq : Inport  Port=2
  Bit Shift1 : hdlsllib/Logic and Bit Operations/Bit Shift  mode=Shift Left Logical  N=Sq_PosIsFrozen
      settings: SourceProductName=HDL Coder  SourceProductBaseCode=HD
  Bit Shift2 : hdlsllib/Logic and Bit Operations/Bit Shift  mode=Shift Left Logical  N=Sq_PosBadGradient
      settings: SourceProductName=HDL Coder  SourceProductBaseCode=HD
  Bit Shift3 : hdlsllib/Logic and Bit Operations/Bit Shift  mode=Shift Left Logical  N=Sq_PosOutOfBounds
      settings: SourceProductName=HDL Coder  SourceProductBaseCode=HD
  Bitwise Operator : simulink/Logic and Bit Operations/Bitwise Operator  logicop=OR  UseBitMask=off  NumInputPorts=4  BitMask=bin2dec('11011001')  BitMaskRealWorld=Stored Integer
  Constant : Constant  Value=checkGradient
  Constant1 : Constant  Value=useAlternativeValue
  Constant2 : Constant  Value=useManualAlternativeValue
  Constant3 : Constant  Value=manualAlternativeValue
  Data Type Conversion1 : DataTypeConversion  OutDataTypeStr=uint8
  Data Type Conversion2 : DataTypeConversion  OutDataTypeStr=uint8
  Data Type Conversion3 : DataTypeConversion  OutDataTypeStr=uint8
  If Action SignalQualifier_PlausibleGradient : Subsystem  TreatAsAtomicUnit=on
  Logical Operator : Logic  Operator=OR  Inputs=3  AllPortsSameDT=off  OutDataTypeStr=boolean
  Logical Operator1 : Logic  AllPortsSameDT=off  OutDataTypeStr=boolean
  Logical Operator2 : Logic  Operator=NOT  Inputs=1  AllPortsSameDT=off  OutDataTypeStr=boolean
  SignalQualifier_FrozenValue : Subsystem
  SignalQualifier_InBounds : Subsystem
  Switch : Switch  Criteria=u2 > Threshold
  Switch1 : Switch  Criteria=u2 > Threshold
  Switch2 : Switch  Criteria=u2 > Threshold
  Unit Delay : UnitDelay  SampleTime=-1  HasFrameUpgradeWarning=on
  lowpass : Subsystem
  Signal_out : Outport  VectorParamsAs1DForOutWhenUnconnected=off
  Signal_Sq_out : Outport  Port=2  VectorParamsAs1DForOutWhenUnconnected=off
  wires:
  Switch1/1 -> Switch2/3
  Logical Operator2/1 -> Switch2/2
  Logical Operator1/1 -> Logical Operator2/1
  Switch2/1 -> Signal_out/1
  Constant3/1 -> Switch1/1
  Constant2/1 -> Switch1/2
  Unit Delay/1 -> Switch/1, Switch1/3
  Switch/1 -> Unit Delay/1
  Constant1/1 -> Logical Operator1/1
  Logical Operator/1 -> Logical Operator1/2, Switch/2  "badSignal"
  Constant/1 -> If Action SignalQualifier_PlausibleGradient/Enable
  Data Type Conversion3/1 -> Bit Shift1/1
  Data Type Conversion2/1 -> Bit Shift3/1
  Data Type Conversion1/1 -> Bit Shift2/1
  Bit Shift2/1 -> Bitwise Operator/1
  Bitwise Operator/1 -> Signal_Sq_out/1
  If Action SignalQualifier_PlausibleGradient/1(BadGradient) -> Logical Operator/1, Data Type Conversion1/1
  SignalQualifier_FrozenValue/1(IsFrozen) -> Data Type Conversion3/1, Logical Operator/3
  SignalQualifier_InBounds/1(IsOutOfBounds) -> Logical Operator/2, Data Type Conversion2/1
  Signal_Sq/1 -> Bitwise Operator/4
  Bit Shift3/1 -> Bitwise Operator/2
  Bit Shift1/1 -> Bitwise Operator/3
  lowpass/1(filtered signal) -> SignalQualifier_InBounds/1(FilteredSignal), If Action SignalQualifier_PlausibleGradient/2(filteredSignal), Switch/3
  Signal/1 -> lowpass/1(signal), If Action SignalQualifier_PlausibleGradient/1(Signal), Switch2/1, SignalQualifier_FrozenValue/1(signal)

== system vd_controller/021_SignalProcessing/214_ManualMode and SimInput/9DFront/Sinus-schwingung ==
  Add : Sum
  Constant : Constant  OutDataTypeStr=single
  Ersatz : Constant  Value=0  OutDataTypeStr=single
  Out1 : Outport  VectorParamsAs1DForOutWhenUnconnected=off
  wires:
  Ersatz/1 -> Add/1
  Add/1 -> Out1/1
  Constant/1 -> Add/2

== system vd_controller/021_SignalProcessing/212_PlausibiltyCheckandSignalMatching/v2oVelocity_Plausibility/EnabledSubsystemAsAlternativeToIfActionPort/If Action SignalQualifier_PlausibleGradient ==
  Signal : Inport
  filteredSignal : Inport  Port=2
  Enable : EnablePort
  SignalQualifier_PlausibleGradient : Subsystem
  BadGradient : Outport  VectorParamsAs1DForOutWhenUnconnected=off
  wires:
  SignalQualifier_PlausibleGradient/1(BadGradient) -> BadGradient/1
  filteredSignal/1 -> SignalQualifier_PlausibleGradient/2(filteredSignal)
  Signal/1 -> SignalQualifier_PlausibleGradient/1(Signal)

== system vd_controller/021_SignalProcessing/212_PlausibiltyCheckandSignalMatching/v2oVelocity_Plausibility/EnabledSubsystemAsAlternativeToIfActionPort/SignalQualifier_FrozenValue ==
  note: step delay:
      | how many steps must
      | the signal be within the
      | range, so that it is
      | detected as frozen
  note: bounds for signalchange
      | standard: 1e-6
  note: Counter which counts the steps, how long the signals are within the threshold
  note: Output
      | =1 if signal is frozen
      | =0 if signal is not frozen
  signal : Inport
  Abs1 : Abs
  Add1 : Sum  Inputs=+-
  Add3 : Sum
  Are the filtered signal and the normal signal near together? : simulink/Logic and Bit Operations/Compare To Constant  relop=<  const=signalBounds  OutDataTypeStr=boolean
  Compare To Constant1 : simulink/Logic and Bit Operations/Compare To Constant  relop=>  const=stepDelay  OutDataTypeStr=boolean
  Data Type Conversion1 : DataTypeConversion
  Data Type Conversion2 : DataTypeConversion
  Product1 : Product
  Unit Delay : UnitDelay  SampleTime=-1  HasFrameUpgradeWarning=on
  Unit Delay1 : UnitDelay  SampleTime=-1  HasFrameUpgradeWarning=on
  IsFrozen : Outport  VectorParamsAs1DForOutWhenUnconnected=off
  wires:
  signal/1 -> Add1/1, Unit Delay/1
  Product1/1 -> Data Type Conversion2/1, Compare To Constant1/1
  Unit Delay1/1 -> Add3/1
  Compare To Constant1/1 -> IsFrozen/1
  Abs1/1 -> Are the filtered signal and the normal signal near together?/1
  Add1/1 -> Abs1/1
  Unit Delay/1 -> Add1/2
  Are the filtered signal and the normal signal near together?/1 -> Data Type Conversion1/1
  Data Type Conversion1/1 -> Add3/2, Product1/2
  Data Type Conversion2/1 -> Unit Delay1/1
  Add3/1 -> Product1/1

== system vd_controller/021_SignalProcessing/212_PlausibiltyCheckandSignalMatching/v2oVelocity_Plausibility/EnabledSubsystemAsAlternativeToIfActionPort/SignalQualifier_InBounds ==
  FilteredSignal : Inport
  Compare To Constant : simulink/Logic and Bit Operations/Compare To Constant  relop=>  const=upperBound  OutDataTypeStr=boolean
  Compare To Constant1 : simulink/Logic and Bit Operations/Compare To Constant  relop=<  const=lowerBound  OutDataTypeStr=boolean
  Logical Operator : Logic  Operator=OR  AllPortsSameDT=off  OutDataTypeStr=boolean
  IsOutOfBounds : Outport  VectorParamsAs1DForOutWhenUnconnected=off
  wires:
  FilteredSignal/1 -> Compare To Constant1/1, Compare To Constant/1
  Compare To Constant/1 -> Logical Operator/1
  Compare To Constant1/1 -> Logical Operator/2
  Logical Operator/1 -> IsOutOfBounds/1

== system vd_controller/021_SignalProcessing/212_PlausibiltyCheckandSignalMatching/v2oVelocity_Plausibility/EnabledSubsystemAsAlternativeToIfActionPort/lowpass ==
  note: Lowpass_alpha is a parameter of the lowpass filter.
      | lowpass_alpha=1  --> no filtering (standard)
      | 0<lowpass_alpha<1   --> inertia of output signal
  signal : Inport
  Add1 : Sum  Inputs=-+
  Add2 : Sum
  Constant : Constant  Value=alpha
  Product : Product
  Unit Delay : UnitDelay  SampleTime=-1  HasFrameUpgradeWarning=on
  filtered signal : Outport  VectorParamsAs1DForOutWhenUnconnected=off
  wires:
  signal/1 -> Add1/2
  Add1/1 -> Product/1
  Add2/1 -> filtered signal/1, Unit Delay/1
  Unit Delay/1 -> Add1/1, Add2/1
  Constant/1 -> Product/2
  Product/1 -> Add2/2

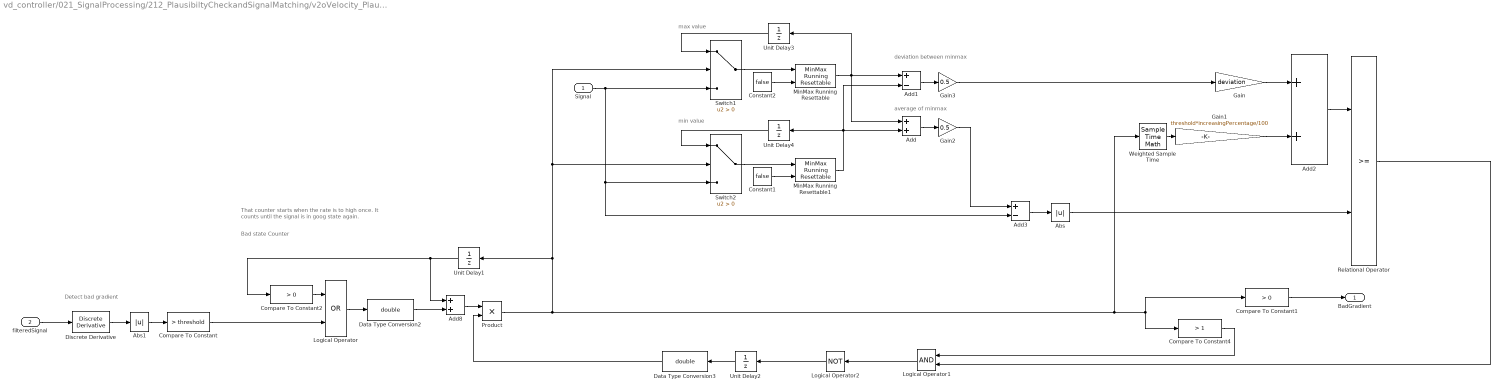
== system vd_controller/021_SignalProcessing/212_PlausibiltyCheckandSignalMatching/v2oVelocity_Plausibility/EnabledSubsystemAsAlternativeToIfActionPort/If Action SignalQualifier_PlausibleGradient/SignalQualifier_PlausibleGradient ==
  note: Detect bad gradient
  note: That counter starts when the rate is to high once.
      | It counts until the signal is in goog state again.
  note: Bad state Counter
  note: max value
  note: min value
  note: average of minmax
  note: deviation between minmax
  Signal : Inport
  filteredSignal : Inport  Port=2
  Abs : Abs
  Abs1 : Abs
  Add : Sum
  Add1 : Sum  Inputs=+-
  Add2 : Sum
  Add3 : Sum  Inputs=+-
  Add8 : Sum  AccumDataTypeStr=double  OutDataTypeStr=double
  Compare To Constant : simulink/Logic and Bit Operations/Compare To Constant  relop=>  const=threshold  OutDataTypeStr=boolean
  Compare To Constant1 : simulink/Logic and Bit Operations/Compare To Constant  relop=>  const=0  OutDataTypeStr=boolean
  Compare To Constant2 : simulink/Logic and Bit Operations/Compare To Constant  relop=>  const=0  OutDataTypeStr=boolean
  Compare To Constant4 : simulink/Logic and Bit Operations/Compare To Constant  relop=>  const=1  OutDataTypeStr=boolean
  Constant1 : Constant  Value=false
  Constant2 : Constant  Value=false
  Data Type Conversion2 : DataTypeConversion  OutDataTypeStr=double
  Data Type Conversion3 : DataTypeConversion  OutDataTypeStr=double
  Discrete Derivative : simulink/Discrete/Discrete Derivative  gainval=1.0  ICPrevScaledInput=0.0  OutMin=[]  OutMax=[]  OutDataType=fixdt(1, 16)  OutScaling=2^-10  DoSatur=off
  Gain : Gain  Gain=deviation
  Gain1 : Gain  Gain=threshold*increasingPercentage/100
  Gain2 : Gain  Gain=0.5
  Gain3 : Gain  Gain=0.5
  Logical Operator : Logic  Operator=OR  AllPortsSameDT=off  OutDataTypeStr=boolean
  Logical Operator1 : Logic  AllPortsSameDT=off  OutDataTypeStr=boolean
  Logical Operator2 : Logic  Operator=NOT  AllPortsSameDT=off  OutDataTypeStr=boolean
  MinMax Running Resettable : simulink/Math Operations/MinMax Running Resettable  Function=max  vinit=0.0
  MinMax Running Resettable1 : simulink/Math Operations/MinMax Running Resettable  Function=min  vinit=0.0
  Product : Product  OutDataTypeStr=double
  Relational Operator : RelationalOperator  OutDataTypeStr=boolean  RndMeth=Simplest
  Switch1 : Switch  Criteria=u2 > Threshold
  Switch2 : Switch  Criteria=u2 > Threshold
  Unit Delay{1..4} (4 alike) : UnitDelay  SampleTime=-1  HasFrameUpgradeWarning=on
  Weighted Sample Time : SampleTimeMath  TsampMathOp=*
  BadGradient : Outport  VectorParamsAs1DForOutWhenUnconnected=off
  wires:
  Unit Delay4/1 -> Switch2/1
  Unit Delay3/1 -> Switch1/1
  Abs/1 -> Relational Operator/2
  Add3/1 -> Abs/1
  Gain2/1 -> Add3/1
  Gain3/1 -> Gain/1
  Add1/1 -> Gain3/1
  Add/1 -> Gain2/1
  MinMax Running Resettable1/1 -> Add/2, Unit Delay4/1, Add1/2
  Switch2/1 -> MinMax Running Resettable1/1
  Constant1/1 -> MinMax Running Resettable1/2
  Constant2/1 -> MinMax Running Resettable/2
  MinMax Running Resettable/1 -> Unit Delay3/1, Add1/1, Add/1
  Switch1/1 -> MinMax Running Resettable/1
  Discrete Derivative/1 -> Abs1/1
  filteredSignal/1 -> Discrete Derivative/1
  Abs1/1 -> Compare To Constant/1
  Compare To Constant/1 -> Logical Operator/2
  Product/1 -> Compare To Constant1/1, Compare To Constant4/1, Weighted Sample Time/1, Unit Delay1/1, Switch2/2, Switch1/2
  Compare To Constant1/1 -> BadGradient/1
  Logical Operator/1 -> Data Type Conversion2/1
  Compare To Constant2/1 -> Logical Operator/1
  Gain/1 -> Add2/1
  Gain1/1 -> Add2/2
  Add2/1 -> Relational Operator/1
  Relational Operator/1 -> Logical Operator1/2
  Logical Operator1/1 -> Logical Operator2/1
  Add8/1 -> Product/1
  Data Type Conversion2/1 -> Add8/2
  Data Type Conversion3/1 -> Product/2
  Signal/1 -> Switch1/3, Add3/2, Switch2/3
  Logical Operator2/1 -> Unit Delay2/1
  Unit Delay1/1 -> Compare To Constant2/1, Add8/1
  Unit Delay2/1 -> Data Type Conversion3/1
  Compare To Constant4/1 -> Logical Operator1/1
  Weighted Sample Time/1 -> Gain1/1
